simulink model "simple_steering"  (R2018a)
settings: Solver=VariableStepAuto  StartTime=0.0  StopTime=10.0  RelTol=1e-3
settings Model: Creator=Emma  LastModifiedBy=Emma

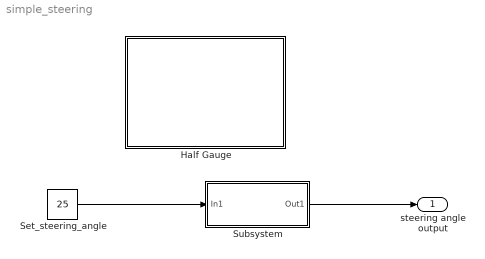
== system simple_steering ==
  Half Gauge : Subsystem  DialogController=hmiCreateDDGDialog  IsWebBlock=on  mask(MWDashboardBlock){webBlockId=38fca1dc-195c-4e31-bb7a-a0a1c0b6e5b9, webBlockType=semicirculargauge, ShowInLibBrowser=on, ShowInitialText=on, HMISrcModelName=simple_steering}
      mask prompts: webBlockId "WebBlock Id"; webBlockType "WebBlock Type"; HMISrcModelName "Source Model"
      mask help: SimulinkHMI:dialogs:SemicircularGaugeDialogDesc
      mask Help: helpview([docroot '/mapfiles/simulink.map'], 'hmi_half_gauge')
      mask Display:
      | if strcmp(get_param(bdroot(gcb),'BlockDiagramType'), 'library')
      |     image([(matlabroot) '/toolbox/simulink/hmi/icons/SemicircularGauge.png']);
      | end
  Set_steering_angle : Constant  Value=25  OutMin=-90  OutMax=90
  Subsystem : Subsystem
  steering angle output : Outport
  wires:
  Set_steering_angle/1 -> Subsystem/1(In1)
  Subsystem/1(Out1) -> steering angle output/1

== system simple_steering/Half Gauge ==

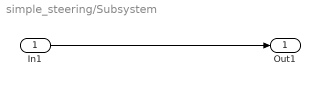
== system simple_steering/Subsystem ==
  In1 : Inport  OutMin=-90  OutMax=90  OutDataTypeStr=uint8
  Out1 : Outport
  wires:
  In1/1 -> Out1/1
